simulink model "Sim_2"  (R2020b)
settings: Solver=VariableStepAuto  StartTime=0.0  StopTime=T_symulacji  RelTol=1e-3
values from neighbouring files (symbols this model uses):
  A_p_kawa = 3.14*r*r    (= 0.005024)    [Projekt2.m]
  A_s_wew = 2*3.14*r*h0_kawy    (= 0.01256)    [Projekt2.m]
  A_s_wew_2 = 2*3.14*r*h_kawy    (= 0.022608)    [Projekt2.m]
  A_s_zew = (2*h-h0_kawy)*2*3.14*r    (= 0.032656)    [Projekt2.m]
  A_s_zew_2 = (2*h-h_kawy)*2*3.14*r    (= 0.022608)    [Projekt2.m]
  alfa_p_kawa = 10    [Projekt2.m]
  alfa_p_s = 10    [Projekt2.m]
  alfa_s_kawa = 250    [Projekt2.m]
  cp_kawy = 4000    [Projekt2.m]
  cp_kawy_2 = 4000    [Projekt2.m]
  cp_s = 800    [Projekt2.m]
  m_kawy = ro_kawy*3.14*r*r*h0_kawy    (= 0.27632)    [Projekt2.m]
  m_mleka = ro_mleka*3.14*r*r*h0_mleka    (= 0.2069888)    [Projekt2.m]
  ro_kawy = 1100    [Projekt2.m]
  ro_kawy_2 = (ro_kawy*h0_kawy+ro_mleka*h0_mleka)/(h0_kawy+h0_mleka)    (= 1068.88888889)    [Projekt2.m]
  ro_s = 2400    [Projekt2.m]
  T0_kawy = 360    [Projekt2.m]
  T0_mleka = 278    [Projekt2.m]
  T0_s = 293    [Projekt2.m]
  Timeop = 500    [Projekt2.m]
  Tp = 293    [Projekt2.m]
  V_kawy = 3.14*r*r*h0_kawy    (= 0.0002512)    [Projekt2.m]
  V_kawy_2 = 3.14*r*r*h_kawy    (= 0.00045216)    [Projekt2.m]
  V_s = 3.14*((r+g)*(r+g)-r*r)*h    (= 4.63464e-05)    [Projekt2.m]
settings Model: Creator=Bartek  LastModifiedBy=Bartek

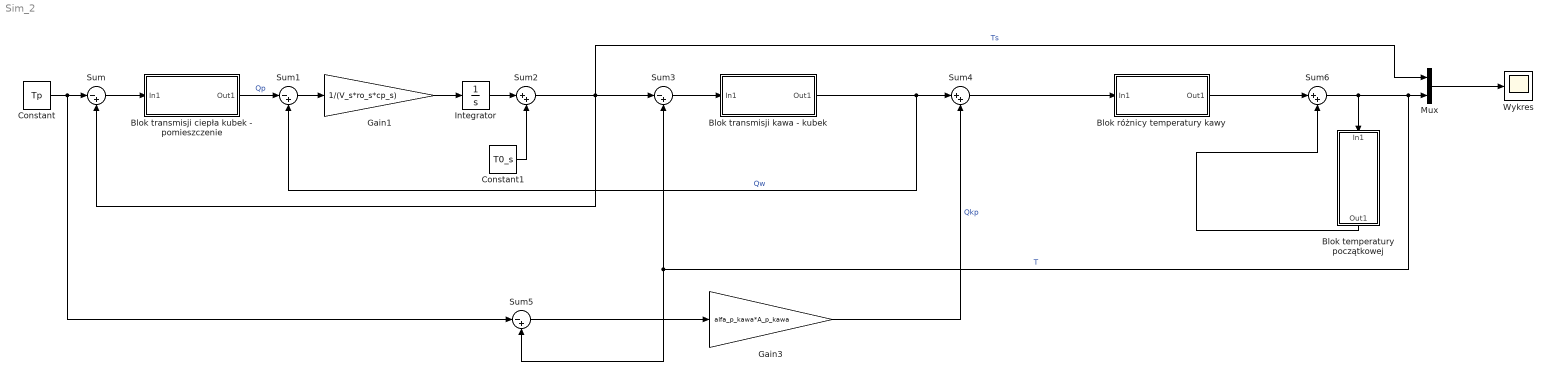
== system Sim_2 ==
  Blok różnicy temperatury kawy : Subsystem
  Blok temperatury początkowej : Subsystem
  Blok transmisji ciepła kubek - pomieszczenie : Subsystem
  "Blok transmisji kawa - kubek " : Subsystem
  Constant : Constant  Value=Tp
  Constant1 : Constant  Value=T0_s
  Gain1 : Gain  Gain=1/(V_s*ro_s*cp_s)
  Gain3 : Gain  Gain=alfa_p_kawa*A_p_kawa
  Integrator : Integrator
  Mux : Mux  Inputs=2
  Sum{,1,3,5} (4 alike) : Sum  Inputs=|-+
  Sum2 : Sum  Inputs=|++
  Sum4 : Sum  Inputs=|++
  Sum6 : Sum  Inputs=|++
  Wykres : Scope
  wires:
  Constant/1 -> Sum5/1, Sum/1
  Sum/1 -> Blok transmisji ciepła kubek - pomieszczenie/1(In1)
  Blok transmisji ciepła kubek - pomieszczenie/1(Out1) -> Sum1/1  "Qp"
  Sum1/1 -> Gain1/1
  Gain1/1 -> Integrator/1
  Integrator/1 -> Sum2/1
  Constant1/1 -> Sum2/2
  Sum2/1 -> Sum/2, Sum3/1, Mux/1  "Ts"
  Sum3/1 -> "Blok transmisji kawa - kubek "/1(In1)
  "Blok transmisji kawa - kubek "/1(Out1) -> Sum4/1, Sum1/2  "Qw"
  Sum5/1 -> Gain3/1
  Gain3/1 -> Sum4/2  "Qkp"
  Sum4/1 -> Blok różnicy temperatury kawy/1(In1)
  Sum6/1 -> Blok temperatury początkowej/1(In1), Mux/2, Sum3/2, Sum5/2  "T"
  Mux/1 -> Wykres/1
  Blok temperatury początkowej/1(Out1) -> Sum6/2
  Blok różnicy temperatury kawy/1(Out1) -> Sum6/1

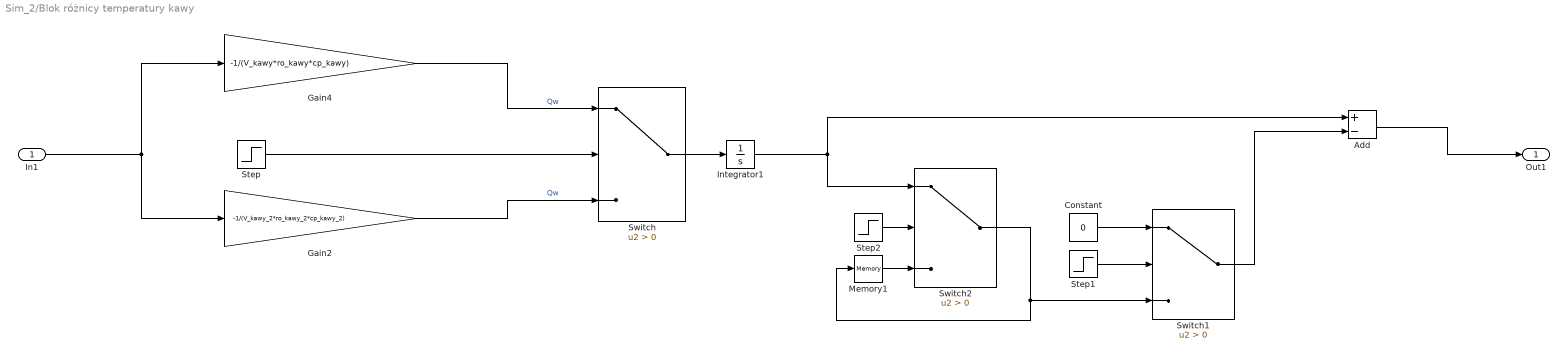
== system Sim_2/Blok różnicy temperatury kawy ==
  In1 : Inport
  Add : Sum  Inputs=+-
  Constant : Constant  Value=0
  Gain2 : Gain  Gain=-1/(V_kawy_2*ro_kawy_2*cp_kawy_2)
  Gain4 : Gain  Gain=-1/(V_kawy*ro_kawy*cp_kawy)
  Integrator1 : Integrator
  Memory1 : Memory
  Step : Step  Time=Timeop  Before=5  After=-1  SampleTime=0
  Step1 : Step  Time=Timeop  Before=5  After=-1  SampleTime=0
  Step2 : Step  Time=Timeop  Before=5  After=-1  SampleTime=0
  Switch : Switch  Criteria=u2 > Threshold
  Switch1 : Switch  Criteria=u2 > Threshold
  Switch2 : Switch  Criteria=u2 > Threshold
  Out1 : Outport
  wires:
  Step/1 -> Switch/2
  In1/1 -> Gain2/1, Gain4/1
  Gain4/1 -> Switch/1  "Qw"
  Gain2/1 -> Switch/3  "Qw"
  Switch/1 -> Integrator1/1
  Switch1/1 -> Add/2
  Step1/1 -> Switch1/2
  Add/1 -> Out1/1
  Step2/1 -> Switch2/2
  Integrator1/1 -> Switch2/1, Add/1
  Switch2/1 -> Switch1/3, Memory1/1
  Memory1/1 -> Switch2/3
  Constant/1 -> Switch1/1

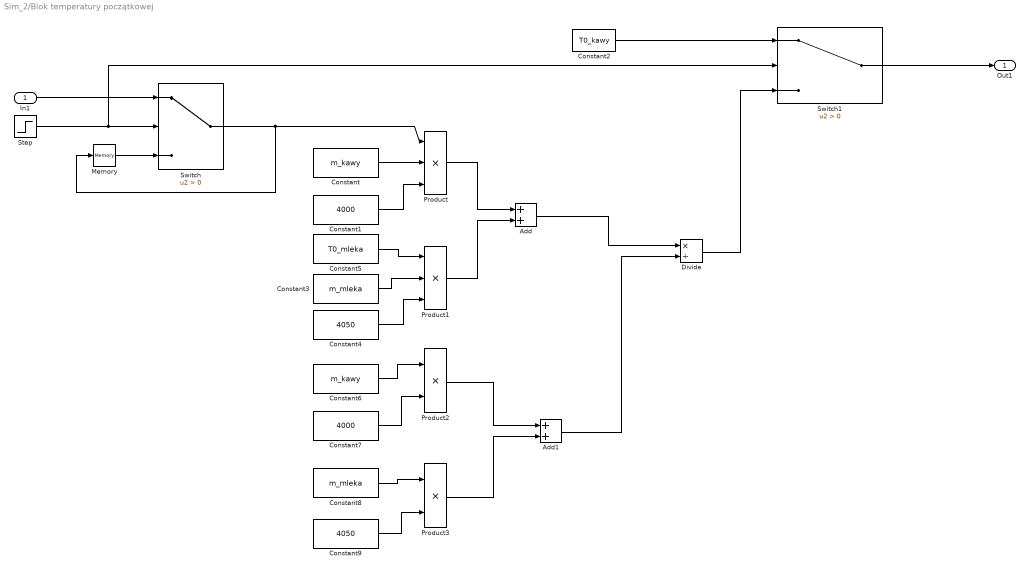
== system Sim_2/Blok temperatury początkowej ==
  In1 : Inport
  Add : Sum
  Add1 : Sum
  Constant : Constant  Value=m_kawy
  Constant1 : Constant  Value=4000
  Constant2 : Constant  Value=T0_kawy
  Constant3 : Constant  Value=m_mleka
  Constant4 : Constant  Value=4050
  Constant5 : Constant  Value=T0_mleka
  Constant6 : Constant  Value=m_kawy
  Constant7 : Constant  Value=4000
  Constant8 : Constant  Value=m_mleka
  Constant9 : Constant  Value=4050
  Divide : Product  Inputs=*/
  Memory : Memory
  Product : Product  Inputs=3
  Product1 : Product  Inputs=3
  Product2 : Product
  Product3 : Product
  Step : Step  Time=Timeop  Before=5  After=-1  SampleTime=0
  Switch : Switch  Criteria=u2 > Threshold
  Switch1 : Switch  Criteria=u2 > Threshold
  Out1 : Outport
  wires:
  Step/1 -> Switch1/2, Switch/2
  In1/1 -> Switch/1
  Switch/1 -> Memory/1, Product/1
  Memory/1 -> Switch/3
  Constant2/1 -> Switch1/1
  Constant1/1 -> Product/3
  Constant/1 -> Product/2
  Constant4/1 -> Product1/3
  Constant3/1 -> Product1/2
  Constant5/1 -> Product1/1
  Product/1 -> Add/1
  Product1/1 -> Add/2
  Add/1 -> Divide/1
  Constant6/1 -> Product2/1
  Constant7/1 -> Product2/2
  Constant8/1 -> Product3/1
  Constant9/1 -> Product3/2
  Product2/1 -> Add1/1
  Product3/1 -> Add1/2
  Add1/1 -> Divide/2
  Divide/1 -> Switch1/3
  Switch1/1 -> Out1/1

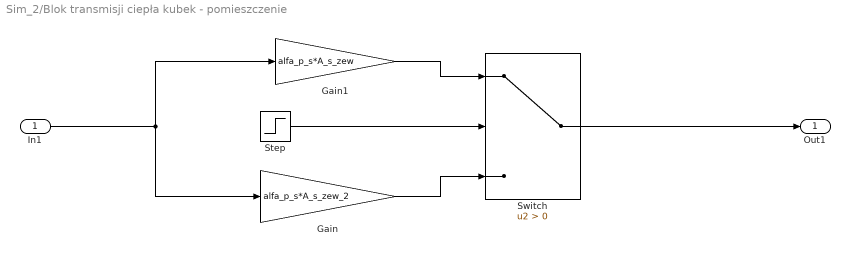
== system Sim_2/Blok transmisji ciepła kubek - pomieszczenie ==
  In1 : Inport
  Gain : Gain  Gain=alfa_p_s*A_s_zew_2
  Gain1 : Gain  Gain=alfa_p_s*A_s_zew
  Step : Step  Time=Timeop  Before=5  After=-1  SampleTime=0
  Switch : Switch  Criteria=u2 > Threshold
  Out1 : Outport
  wires:
  Step/1 -> Switch/2
  Gain/1 -> Switch/3
  In1/1 -> Gain/1, Gain1/1
  Gain1/1 -> Switch/1
  Switch/1 -> Out1/1

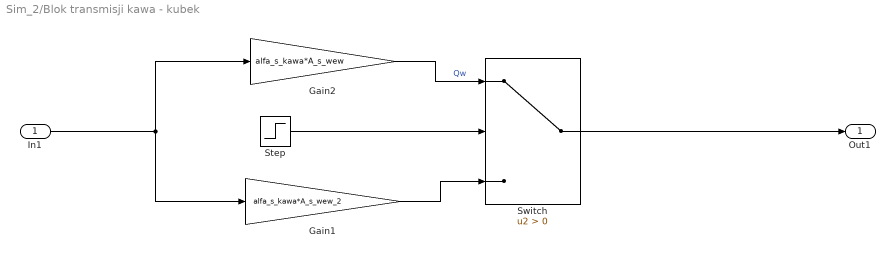
== system Sim_2/Blok transmisji kawa - kubek  ==
  In1 : Inport
  Gain1 : Gain  Gain=alfa_s_kawa*A_s_wew_2
  Gain2 : Gain  Gain=alfa_s_kawa*A_s_wew
  Step : Step  Time=Timeop  Before=5  After=-1  SampleTime=0
  Switch : Switch  Criteria=u2 > Threshold
  Out1 : Outport
  wires:
  Step/1 -> Switch/2
  Gain1/1 -> Switch/3
  In1/1 -> Gain1/1, Gain2/1
  Switch/1 -> Out1/1
  Gain2/1 -> Switch/1  "Qw"
